simulink model "filterChain"  (R2016a)
settings: Solver=VariableStepAuto  StartTime=0.0  StopTime=2e-3  RelTol=1e-3
values from neighbouring files (symbols this model uses):
  f = [fp fs]    [cicSimu.m]
  L = 110    [cicSimu.m]
  Mf = [Mp zeros(1,length(fr)-length(Mp))]    [cicSimu.m]
undefined symbols (not defined in the file or in its folder): fir2
libraries: xbsIndex_r4 x35, components x14, dspsrcs4 x1
settings Model: Creator=raphael.frey  LastModifiedBy=raphael.frey

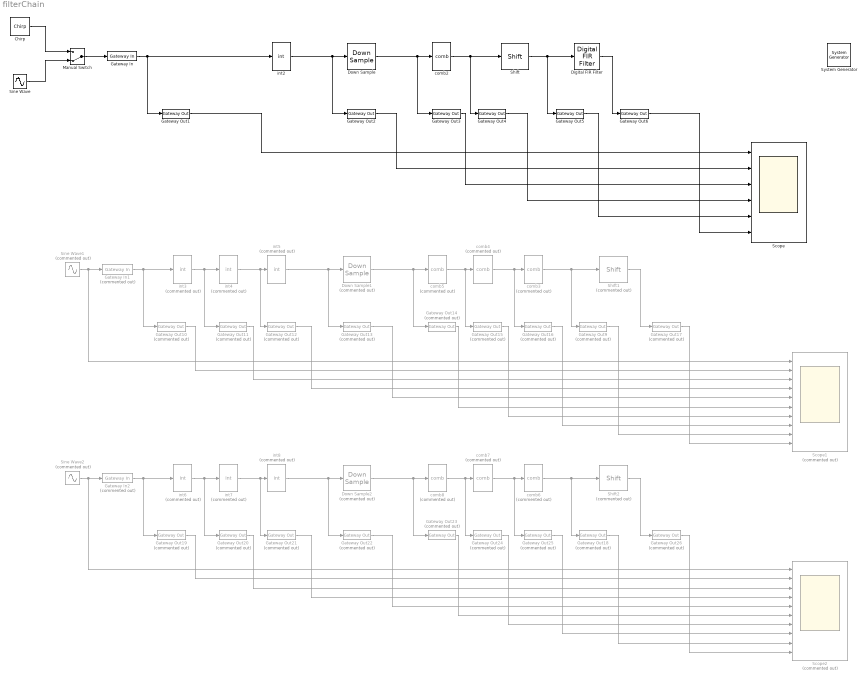
== system filterChain ==
  " System Generator" : xbsIndex_r4/ System Generator  Tag=genX  xilinxfamily=zynq  part=xc7z010  speed=-1  package=clg400  synthesis_tool=Vivado  clock_wrapper=Clock Enables  directory=./netlist  proj_type=Vivado  Synth_file=Vivado Synthesis Defaults  Impl_file=Vivado Implementation Defaults  testbench=off  simulink_period=8e-9  sysclk_period=8  dcm_input_clock_period=10  incr_netlist=off  trim_vbits=Everywhere in SubSystem  dbl_ovrd=According to Block Masks  core_generation=According to Block Masks  run_coregen=off  deprecated_control=off  eval_field=0  block_type=sysgen
  Chirp : dspsrcs4/Chirp  sweep=Linear  mode=Unidirectional  f0=1000  f1=384e3  t1=0.01  Tsweep=1  phase=0  Ts=8e-9  spf=1  datatype=Double  OutputFrames=off
  Digital FIR Filter : xbsIndex_r4/Digital FIR Filter  coeff_source=off  coefficientvector=fir2(L,f,Mf)  coeff_calulate=on  coefficient_width=2  coefficient_fractional_bits=0  interpolation_filter_rate=1  decimation_filter_rate=1  fda_coefficientvector=[-0.0024 -0.0042 0.0095 0.0200 -0.0380 -0.0696 0.1374 0.4472 0.4472 0.1374 -0.0696 -0.0380 0.0200 0.0095 -0.0042 -0.0024]  simulation_type=fast_sim  simulation_model=sysgen:fir_macro  block_type=fir_macro
  Down Sample : xbsIndex_r4/Down Sample  sample_ratio=650  sample_phase="Last Value of Frame  (most efficient)"  en=off  rst=off  latency=1  dbl_ovrd=off  block_type=dsamp
  Down Sample1 : xbsIndex_r4/Down Sample  Commented=on  sample_ratio=2500  sample_phase="Last Value of Frame  (most efficient)"  en=off  rst=off  latency=1  dbl_ovrd=off  block_type=dsamp
  Down Sample2 : xbsIndex_r4/Down Sample  Commented=on  sample_ratio=2500  sample_phase="Last Value of Frame  (most efficient)"  en=off  rst=off  latency=1  dbl_ovrd=off  block_type=dsamp
  Gateway In : xbsIndex_r4/Gateway In  gui_display_data_type=Fixed-point  arith_type="Signed  (2's comp)"  n_bits=14  bin_pt=0  preci_type=Single  exp_width=8  frac_width=24  rows=1  columns=1  quantization=Truncate  overflow=Wrap  period=8e-9  UseAsADC=off  ADCChannel='1'  interface=None  automatic_assignment=on  address_offset=hex2dec('00')  intf_name=''  intf_description=''  default_value=0  timing_constraint=None  locs_specified=off  LOCs={}  io_standard={}  inherit_from_input=off  hdl_port=on  dbl_ovrd=off  block_type=gatewayin
  Gateway In1 : xbsIndex_r4/Gateway In  Commented=on  gui_display_data_type=Fixed-point  arith_type="Signed  (2's comp)"  n_bits=14  bin_pt=0  preci_type=Single  exp_width=8  frac_width=24  rows=1  columns=1  quantization=Truncate  overflow=Wrap  period=8e-9  UseAsADC=off  ADCChannel='1'  interface=None  automatic_assignment=on  address_offset=hex2dec('00')  intf_name=''  intf_description=''  default_value=0  timing_constraint=None  locs_specified=off  LOCs={}  io_standard={}  inherit_from_input=off  hdl_port=on  dbl_ovrd=off  block_type=gatewayin
  Gateway In2 : xbsIndex_r4/Gateway In  Commented=on  gui_display_data_type=Fixed-point  arith_type="Signed  (2's comp)"  n_bits=14  bin_pt=0  preci_type=Single  exp_width=8  frac_width=24  rows=1  columns=1  quantization=Truncate  overflow=Wrap  period=8e-9  UseAsADC=off  ADCChannel='1'  interface=None  automatic_assignment=on  address_offset=hex2dec('00')  intf_name=''  intf_description=''  default_value=0  timing_constraint=None  locs_specified=off  LOCs={}  io_standard={}  inherit_from_input=off  hdl_port=on  dbl_ovrd=off  block_type=gatewayin
  Gateway Out{1..6} (6 alike) : xbsIndex_r4/Gateway Out  inherit_from_input=off  hdl_port=on  rows=1  columns=1  UseAsDAC=off  DACChannel='1'  interface=None  automatic_assignment=on  address_offset=hex2dec('00')  intf_name=''  intf_description=''  timing_constraint=None  locs_specified=off  LOCs={}  io_standard={}  block_type=gatewayout
  Gateway Out{9..26} (18 alike) : xbsIndex_r4/Gateway Out  Commented=on  inherit_from_input=off  hdl_port=on  rows=1  columns=1  UseAsDAC=off  DACChannel='1'  interface=None  automatic_assignment=on  address_offset=hex2dec('00')  intf_name=''  intf_description=''  timing_constraint=None  locs_specified=off  LOCs={}  io_standard={}  block_type=gatewayout
  Manual Switch : ManualSwitch  CurrentSetting=0
  Scope : Scope  NumInputPorts=6
  Scope1 : Scope  Commented=on  NumInputPorts=10
  Scope2 : Scope  Commented=on  NumInputPorts=10
  Shift : xbsIndex_r4/Shift  shift_dir=Right  shift_bits=9  en=off  latency=0  precision=User Defined  arith_type="Signed  (2's comp)"  n_bits=16  bin_pt=0  quantization=Truncate  overflow=Wrap  dbl_ovrd=off  block_type=shift
  Shift1 : xbsIndex_r4/Shift  Commented=on  shift_dir=Right  shift_bits=34  en=off  latency=0  precision=User Defined  arith_type="Signed  (2's comp)"  n_bits=16  bin_pt=0  quantization=Truncate  overflow=Wrap  dbl_ovrd=off  block_type=shift
  Shift2 : xbsIndex_r4/Shift  Commented=on  shift_dir=Right  shift_bits=34  en=off  latency=0  precision=User Defined  arith_type="Signed  (2's comp)"  n_bits=16  bin_pt=0  quantization=Truncate  overflow=Wrap  dbl_ovrd=off  block_type=shift
  Sine Wave : Sin  Amplitude=2^12  Frequency=2*pi*1e3  Samples=100  SampleTime=0
  Sine Wave1 : Sin  Commented=on  Amplitude=2^12  Frequency=2*pi*1e3  Samples=100  SampleTime=0
  Sine Wave2 : Sin  Commented=on  Amplitude=2^12  Frequency=2*pi*1e3  Samples=100  SampleTime=0
  comb2 : components/comb
      link override AddSub: mode=Subtraction  use_carryin=off  use_carryout=off  en=off  latency=0  precision=User Defined  arith_type="Signed  (2's comp)"  n_bits=24  bin_pt=0  quantization=Truncate  overflow=Wrap  use_behavioral_HDL=off  hw_selection=Fabric  pipelined=off  dbl_ovrd=off
  comb3 : components/comb  Commented=on
      link override AddSub: mode=Subtraction  use_carryin=off  use_carryout=off  en=off  latency=0  precision=User Defined  arith_type="Signed  (2's comp)"  n_bits=53  bin_pt=0  quantization=Truncate  overflow=Wrap  use_behavioral_HDL=off  hw_selection=Fabric  pipelined=off  dbl_ovrd=off
  comb4 : components/comb  Commented=on
      link override AddSub: mode=Subtraction  use_carryin=off  use_carryout=off  en=off  latency=0  precision=User Defined  arith_type="Signed  (2's comp)"  n_bits=53  bin_pt=0  quantization=Truncate  overflow=Wrap  use_behavioral_HDL=off  hw_selection=Fabric  pipelined=off  dbl_ovrd=off
  comb5 : components/comb  Commented=on
      link override AddSub: mode=Subtraction  use_carryin=off  use_carryout=off  en=off  latency=0  precision=User Defined  arith_type="Signed  (2's comp)"  n_bits=53  bin_pt=0  quantization=Truncate  overflow=Wrap  use_behavioral_HDL=off  hw_selection=Fabric  pipelined=off  dbl_ovrd=off
  comb6 : components/comb  Commented=on
      link override AddSub: mode=Subtraction  use_carryin=off  use_carryout=off  en=off  latency=0  precision=User Defined  arith_type="Signed  (2's comp)"  n_bits=53  bin_pt=0  quantization=Truncate  overflow=Wrap  use_behavioral_HDL=off  hw_selection=Fabric  pipelined=off  dbl_ovrd=off
  comb7 : components/comb  Commented=on
      link override AddSub: mode=Subtraction  use_carryin=off  use_carryout=off  en=off  latency=0  precision=User Defined  arith_type="Signed  (2's comp)"  n_bits=53  bin_pt=0  quantization=Truncate  overflow=Wrap  use_behavioral_HDL=off  hw_selection=Fabric  pipelined=off  dbl_ovrd=off
  comb8 : components/comb  Commented=on
      link override AddSub: mode=Subtraction  use_carryin=off  use_carryout=off  en=off  latency=0  precision=User Defined  arith_type="Signed  (2's comp)"  n_bits=53  bin_pt=0  quantization=Truncate  overflow=Wrap  use_behavioral_HDL=off  hw_selection=Fabric  pipelined=off  dbl_ovrd=off
  int2 : components/int
      link override AddSub: mode=Addition  use_carryin=off  use_carryout=off  en=off  latency=0  precision=User Defined  arith_type="Signed  (2's comp)"  n_bits=24  bin_pt=0  quantization=Truncate  overflow=Wrap  use_behavioral_HDL=off  hw_selection=Fabric  pipelined=off  dbl_ovrd=off
  int3 : components/int  Commented=on
      link override AddSub: mode=Addition  use_carryin=off  use_carryout=off  en=off  latency=0  precision=User Defined  arith_type="Signed  (2's comp)"  n_bits=53  bin_pt=0  quantization=Truncate  overflow=Wrap  use_behavioral_HDL=off  hw_selection=Fabric  pipelined=off  dbl_ovrd=off
  int4 : components/int  Commented=on
      link override AddSub: mode=Addition  use_carryin=off  use_carryout=off  en=off  latency=0  precision=User Defined  arith_type="Signed  (2's comp)"  n_bits=53  bin_pt=0  quantization=Truncate  overflow=Wrap  use_behavioral_HDL=off  hw_selection=Fabric  pipelined=off  dbl_ovrd=off
  int5 : components/int  Commented=on
      link override AddSub: mode=Addition  use_carryin=off  use_carryout=off  en=off  latency=0  precision=User Defined  arith_type="Signed  (2's comp)"  n_bits=53  bin_pt=0  quantization=Truncate  overflow=Wrap  use_behavioral_HDL=off  hw_selection=Fabric  pipelined=off  dbl_ovrd=off
  int6 : components/int  Commented=on
      link override AddSub: mode=Addition  use_carryin=off  use_carryout=off  en=off  latency=0  precision=User Defined  arith_type="Signed  (2's comp)"  n_bits=53  bin_pt=0  quantization=Truncate  overflow=Wrap  use_behavioral_HDL=off  hw_selection=Fabric  pipelined=off  dbl_ovrd=off
  int7 : components/int  Commented=on
      link override AddSub: mode=Addition  use_carryin=off  use_carryout=off  en=off  latency=0  precision=User Defined  arith_type="Signed  (2's comp)"  n_bits=53  bin_pt=0  quantization=Truncate  overflow=Wrap  use_behavioral_HDL=off  hw_selection=Fabric  pipelined=off  dbl_ovrd=off
  int8 : components/int  Commented=on
      link override AddSub: mode=Addition  use_carryin=off  use_carryout=off  en=off  latency=0  precision=User Defined  arith_type="Signed  (2's comp)"  n_bits=53  bin_pt=0  quantization=Truncate  overflow=Wrap  use_behavioral_HDL=off  hw_selection=Fabric  pipelined=off  dbl_ovrd=off
  wires:
  Gateway In/1 -> int2/1, Gateway Out1/1
  Down Sample/1 -> Gateway Out3/1, comb2/1
  comb2/1 -> Gateway Out4/1, Shift/1
  int2/1 -> Gateway Out2/1, Down Sample/1
  Shift/1 -> Gateway Out5/1, Digital FIR Filter/1
  Sine Wave1/1 -> Scope1/1, Gateway In1/1
  Gateway In1/1 -> int3/1, Gateway Out10/1
  comb3/1 -> Gateway Out9/1, Shift1/1
  int3/1 -> Gateway Out11/1, int4/1
  int4/1 -> Gateway Out12/1, int5/1
  Down Sample1/1 -> Gateway Out14/1, comb5/1
  comb5/1 -> Gateway Out15/1, comb4/1
  comb4/1 -> Gateway Out16/1, comb3/1
  int5/1 -> Gateway Out13/1, Down Sample1/1
  Gateway Out10/1 -> Scope1/2
  Gateway Out11/1 -> Scope1/3
  Gateway Out12/1 -> Scope1/4
  Gateway Out13/1 -> Scope1/5
  Gateway Out14/1 -> Scope1/6
  Gateway Out15/1 -> Scope1/7
  Gateway Out16/1 -> Scope1/8
  Gateway Out9/1 -> Scope1/9
  Shift1/1 -> Gateway Out17/1
  Gateway Out17/1 -> Scope1/10
  Sine Wave2/1 -> Scope2/1, Gateway In2/1
  Gateway In2/1 -> int6/1, Gateway Out19/1
  comb6/1 -> Gateway Out18/1, Shift2/1
  int6/1 -> Gateway Out20/1, int7/1
  int7/1 -> Gateway Out21/1, int8/1
  Down Sample2/1 -> Gateway Out23/1, comb8/1
  comb8/1 -> Gateway Out24/1, comb7/1
  comb7/1 -> Gateway Out25/1, comb6/1
  int8/1 -> Gateway Out22/1, Down Sample2/1
  Gateway Out19/1 -> Scope2/2
  Gateway Out20/1 -> Scope2/3
  Gateway Out21/1 -> Scope2/4
  Gateway Out22/1 -> Scope2/5
  Gateway Out23/1 -> Scope2/6
  Gateway Out24/1 -> Scope2/7
  Gateway Out25/1 -> Scope2/8
  Gateway Out18/1 -> Scope2/9
  Shift2/1 -> Gateway Out26/1
  Gateway Out26/1 -> Scope2/10
  Digital FIR Filter/1 -> Gateway Out6/1
  Sine Wave/1 -> Manual Switch/2
  Chirp/1 -> Manual Switch/1
  Manual Switch/1 -> Gateway In/1
  Gateway Out6/1 -> Scope/6
  Gateway Out5/1 -> Scope/5
  Gateway Out4/1 -> Scope/4
  Gateway Out3/1 -> Scope/3
  Gateway Out2/1 -> Scope/2
  Gateway Out1/1 -> Scope/1
